simulink model "arch"  (R2016b)
settings: Solver=VariableStepAuto  StartTime=0.0  StopTime=10.0  RelTol=1e-3
settings Model: Creator=fabia  LastModifiedBy=fabia

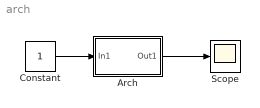
== system arch ==
  Arch : Subsystem
  Constant : Constant
  Scope : Scope
  wires:
  Constant/1 -> Arch/1(In1)
  Arch/1(Out1) -> Scope/1

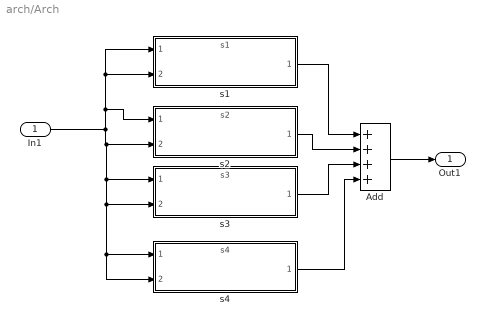
== system arch/Arch ==
  In1 : Inport
  Add : Sum  Inputs=++++
  s1 : ModelReference  ModelNameDialog=s1.slx  SimulationMode=Normal  ModelReferenceVersion=1.2
  s2 : ModelReference  ModelNameDialog=s2.slx  SimulationMode=Normal  ModelReferenceVersion=1.1
  s3 : ModelReference  ModelNameDialog=s3.slx  SimulationMode=Normal  ModelReferenceVersion=1.1
  s4 : ModelReference  ModelNameDialog=s4.slx  SimulationMode=Normal  ModelReferenceVersion=1.1
  Out1 : Outport
  wires:
  s1/1 -> Add/1
  s4/1 -> Add/4
  Add/1 -> Out1/1
  In1/1 -> s4/2, s4/1, s3/2, s3/1, s2/2, s2/1, s1/2, s1/1
  s2/1 -> Add/2
  s3/1 -> Add/3
